simulink library "PhD_Library"  (R2018a)
settings: Solver=VariableStepAuto  StartTime=0.0  StopTime=10.0  RelTol=1e-3
values from neighbouring files (symbols this model uses):
  Ts = Ts_c    (= 1e-07)    [PlantStateEquations_abc_Script.m]
undefined symbols (not defined in the file or in its folder): D1, Delta, DiscIntNeverNeededParam, ESS, f_LPF_noise, fcutouti, fcutoutv, fn, fsw, Iap, Kp, PCC, Sn, tctrl, Ti, Ts_control, Ts_PWM, Uabp, Uanp, WT, X, zeta
libraries: $bdroot x84, powerlib_meascontrol x59, powerlib x56, peTransforms x32, cstblocks x2, simulink x2
(part 4 of 5)

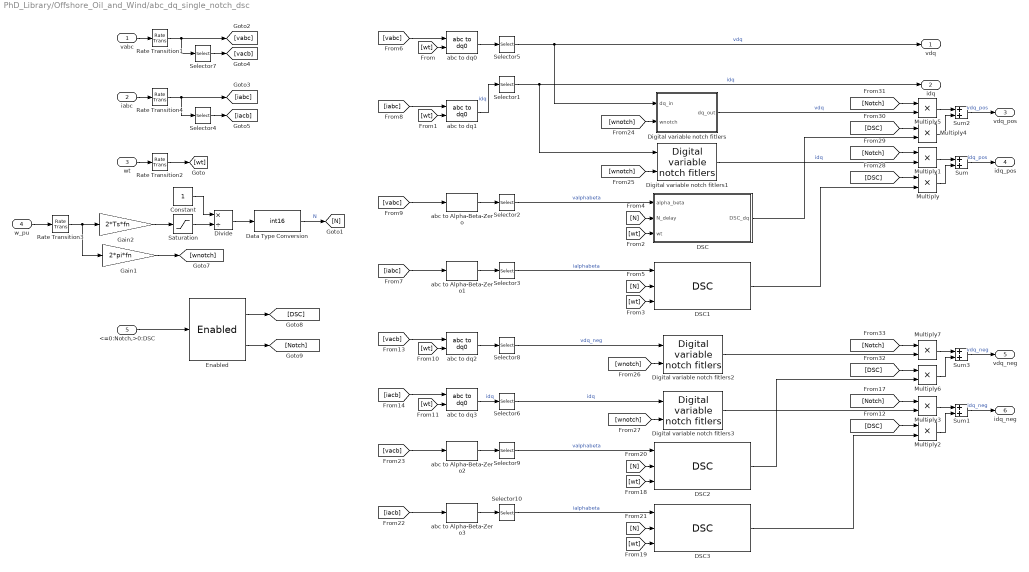
== system PhD_Library/Offshore_Oil_and_Wind/abc_dq_single_notch_dsc ==
  vabc : Inport
  iabc : Inport  Port=2
  wt : Inport  Port=3
  w_pu : Inport  Port=4
  <=0:Notch,>0:DSC : Inport  Port=5
  Constant : Constant
  DSC : Subsystem
  DSC1 : $bdroot/Offshore_Oil_and_Wind/abc_dq_single_notch_dsc/DSC
  DSC2 : $bdroot/Offshore_Oil_and_Wind/abc_dq_single_notch_dsc/DSC
  DSC3 : $bdroot/Offshore_Oil_and_Wind/abc_dq_single_notch_dsc/DSC
  Data Type Conversion : DataTypeConversion  OutDataTypeStr=int16  RndMeth=Round  SaturateOnIntegerOverflow=on
  Digital variable notch fitlers : Subsystem
  Digital variable notch fitlers1 : $bdroot/Offshore_Oil_and_Wind/abc_dq_single_notch_dsc/Digital variable notch fitlers
  Digital variable notch fitlers2 : $bdroot/Offshore_Oil_and_Wind/abc_dq_single_notch_dsc/Digital variable notch fitlers
  Digital variable notch fitlers3 : $bdroot/Offshore_Oil_and_Wind/abc_dq_single_notch_dsc/Digital variable notch fitlers
  Divide : Product  Inputs=*/
  Enabled : $bdroot/Offshore_Oil_and_Wind/Enabled
  Gain1 : Gain  Gain=2*pi*fn
  Gain2 : Gain  Gain=2*Ts*fn
  Multiply{,1..7} (8 alike) : Product
  Rate Transition1 : RateTransition  OutPortSampleTime=Ts
  Rate Transition2 : RateTransition  OutPortSampleTime=Ts
  Rate Transition3 : RateTransition  InitialCondition=1  OutPortSampleTime=Ts
  Rate Transition4 : RateTransition  OutPortSampleTime=Ts
  Saturation : Saturate  UpperLimit=inf  LowerLimit=0.000001
  Selector{1..3,5..6,8..10} (8 alike) : Selector  InputPortWidth=3  IndexOptions=Index vector (dialog)  Indices=[1 2]  OutputSizes=1
  Selector4 : Selector  InputPortWidth=3  IndexOptions=Index vector (dialog)  Indices=[1 3 2]  OutputSizes=1
  Selector7 : Selector  InputPortWidth=3  IndexOptions=Index vector (dialog)  Indices=[1 3 2]  OutputSizes=1
  Sum{,1..3} (4 alike) : Sum
  abc to Alpha-Beta-Zero{,1..3} (4 alike) : powerlib_meascontrol/Transformations/abc to Alpha-Beta-Zero
      settings: SourceProductName=Simscape Power Systems
  abc to dq{0..3} (4 alike) : powerlib_meascontrol/Transformations/abc to dq0  Alignment=90 degrees behind phase A axis
  vdq : Outport
  idq : Outport  Port=2
  vdq_pos : Outport  Port=3
  idq_pos : Outport  Port=4
  vdq_neg : Outport  Port=5
  idq_neg : Outport  Port=6
  wires:
  wt/1 -> Rate Transition2/1
  abc to dq1/1 -> Selector1/1  "idq"
  Selector5/1 -> Digital variable notch fitlers/1(dq_in), vdq/1  "vdq"
  abc to dq0/1 -> Selector5/1
  Selector1/1 -> Digital variable notch fitlers1/1, idq/1  "idq"
  abc to Alpha-Beta-Zero/1 -> Selector2/1
  abc to Alpha-Beta-Zero1/1 -> Selector3/1
  DSC/1(DSC_dq) -> Multiply4/2
  Selector3/1 -> DSC1/1  "ialphabeta"
  [vabc] -> abc to dq0/1
  [iabc] -> abc to dq1/1
  vabc/1 -> Rate Transition1/1
  iabc/1 -> Rate Transition4/1
  Selector2/1 -> DSC/1(alpha_beta)  "valphabeta"
  Digital variable notch fitlers/1(dq_out) -> Multiply5/2  "vdq"
  Digital variable notch fitlers1/1 -> Multiply1/2  "idq"
  DSC1/1 -> Multiply/2
  Sum2/1 -> vdq_pos/1  "vdq_pos"
  Sum/1 -> idq_pos/1  "idq_pos"
  Rate Transition2/1 -> [wt]
  [wt] -> abc to dq0/2
  [wt] -> abc to dq1/2
  [wt] -> DSC/3(wt)
  [wt] -> DSC1/3
  [N] -> DSC/2(N_delay)
  [N] -> DSC1/2
  Data Type Conversion/1 -> [N]  "N"
  Rate Transition1/1 -> Selector7/1, [vabc]
  Selector7/1 -> [vacb]
  Rate Transition4/1 -> Selector4/1, [iabc]
  Selector4/1 -> [iacb]
  [vabc] -> abc to Alpha-Beta-Zero/1
  [iabc] -> abc to Alpha-Beta-Zero1/1
  [wt] -> abc to dq3/2
  abc to dq2/1 -> Selector8/1
  Selector8/1 -> Digital variable notch fitlers2/1  "vdq_neg"
  [vacb] -> abc to dq2/1
  [wt] -> abc to dq2/2
  abc to dq3/1 -> Selector6/1  "idq"
  [iacb] -> abc to dq3/1
  Sum3/1 -> vdq_neg/1  "vdq_neg"
  Sum1/1 -> idq_neg/1  "idq_neg"
  Digital variable notch fitlers2/1 -> Multiply7/2
  Selector6/1 -> Digital variable notch fitlers3/1  "idq"
  Digital variable notch fitlers3/1 -> Multiply3/2
  abc to Alpha-Beta-Zero3/1 -> Selector10/1
  Selector10/1 -> DSC3/1  "ialphabeta"
  abc to Alpha-Beta-Zero2/1 -> Selector9/1
  [iacb] -> abc to Alpha-Beta-Zero3/1
  [wt] -> DSC2/3
  [vacb] -> abc to Alpha-Beta-Zero2/1
  DSC2/1 -> Multiply6/2
  Selector9/1 -> DSC2/1  "valphabeta"
  [N] -> DSC3/2
  [N] -> DSC2/2
  DSC3/1 -> Multiply2/2
  [wt] -> DSC3/3
  Gain2/1 -> Saturation/1
  Saturation/1 -> Divide/2
  Constant/1 -> Divide/1
  Rate Transition3/1 -> Gain1/1, Gain2/1
  Divide/1 -> Data Type Conversion/1
  w_pu/1 -> Rate Transition3/1
  Gain1/1 -> [wnotch]
  [wnotch] -> Digital variable notch fitlers/2(wnotch)
  [wnotch] -> Digital variable notch fitlers1/2
  [wnotch] -> Digital variable notch fitlers2/2
  [wnotch] -> Digital variable notch fitlers3/2
  <=0:Notch,>0:DSC/1 -> Enabled/1
  Enabled/1 -> [DSC]
  Enabled/2 -> [Notch]
  [DSC] -> Multiply/1
  [Notch] -> Multiply1/1
  Multiply1/1 -> Sum/1
  Multiply/1 -> Sum/2
  [Notch] -> Multiply3/1
  [DSC] -> Multiply2/1
  Multiply3/1 -> Sum1/1
  Multiply2/1 -> Sum1/2
  [Notch] -> Multiply5/1
  Multiply4/1 -> Sum2/2
  [DSC] -> Multiply4/1
  Multiply5/1 -> Sum2/1
  [Notch] -> Multiply7/1
  Multiply6/1 -> Sum3/2
  [DSC] -> Multiply6/1
  Multiply7/1 -> Sum3/1

== system PhD_Library/Offshore_Oil_and_Wind/abc_dq_with_AMA ==
  vabc : Inport
  iabc : Inport  Port=2
  wt : Inport  Port=3
  w_pu : Inport  Port=4
  AMA with retrieval pointer driven buffer{1..4} (4 alike) : $bdroot/Adaptive Moving Averages/AMA with retrieval pointer driven buffer  NbSize=1/(2*fmin*Ts)  Ts=Ts
  Bus Creator : BusCreator  Inputs=4
  Constant : Constant  Value=2*Ts
  Constant1 : Constant
  Demux : Demux  Outputs=2
  Demux1 : Demux  Outputs=2
  Digital first order LPF : $bdroot/Offshore_Oil_and_Wind/Digital first order LPF  Ts=Ts  fcutout=fcutoutv
  Digital first order LPF1 : $bdroot/Offshore_Oil_and_Wind/Digital first order LPF  Ts=Ts  fcutout=fcutouti
  Divide : Product  Inputs=*/
  Gain : Gain  Gain=fn
  Mux : Mux  Inputs=2
  Mux1 : Mux  Inputs=2
  Product : Product
  Rate Transition1 : RateTransition  OutPortSampleTime=Ts
  Rate Transition2 : RateTransition  OutPortSampleTime=Ts
  Rate Transition3 : RateTransition  InitialCondition=1  OutPortSampleTime=Ts
  Rate Transition4 : RateTransition  OutPortSampleTime=Ts
  Saturation : Saturate  UpperLimit=fmax  LowerLimit=fmin
  Selector4 : Selector  InputPortWidth=3  IndexOptions=Index vector (dialog)  Indices=[1 2]  OutputSizes=1
  Selector5 : Selector  InputPortWidth=3  IndexOptions=Index vector (dialog)  Indices=[1 2]  OutputSizes=1
  Terminator{1..8} (8 alike) : Terminator
  abc to dq0 : powerlib_meascontrol/Transformations/abc to dq0  Alignment=90 degrees behind phase A axis
  abc to dq1 : powerlib_meascontrol/Transformations/abc to dq0  Alignment=90 degrees behind phase A axis
  vdq : Outport
  idq : Outport  Port=2
  m : Outport  Port=3
  wires:
  Digital first order LPF/1 -> Demux/1  "vdq"
  abc to dq1/1 -> Selector4/1
  Mux1/1 -> Bus Creator/4, idq/1  "idq"
  Selector5/1 -> Digital first order LPF/1, Bus Creator/1  "vdq_unfilt"
  Rate Transition1/1 -> abc to dq0/1
  Rate Transition2/1 -> abc to dq0/2, abc to dq1/2
  Selector4/1 -> Bus Creator/2, Digital first order LPF1/1  "idq_unfilt"
  Rate Transition4/1 -> abc to dq1/1
  abc to dq0/1 -> Selector5/1
  Bus Creator/1 -> m/1
  Mux/1 -> Bus Creator/3, vdq/1  "vdq"
  wt/1 -> Rate Transition2/1
  vabc/1 -> Rate Transition1/1
  iabc/1 -> Rate Transition4/1
  AMA with retrieval pointer driven buffer1/3 -> Terminator2/1
  AMA with retrieval pointer driven buffer1/2 -> Terminator3/1
  w_pu/1 -> Rate Transition3/1
  Rate Transition3/1 -> Gain/1
  Gain/1 -> Saturation/1
  Saturation/1 -> Product/1
  Constant/1 -> Product/2
  Product/1 -> Divide/2
  Constant1/1 -> Divide/1
  Divide/1 -> [N]
  Demux/1 -> AMA with retrieval pointer driven buffer2/1
  Demux/2 -> AMA with retrieval pointer driven buffer1/1
  AMA with retrieval pointer driven buffer2/3 -> Terminator4/1
  AMA with retrieval pointer driven buffer2/2 -> Terminator5/1
  AMA with retrieval pointer driven buffer2/1 -> Mux/1
  AMA with retrieval pointer driven buffer1/1 -> Mux/2  "vdq"
  AMA with retrieval pointer driven buffer3/1 -> Mux1/2  "vdq"
  AMA with retrieval pointer driven buffer4/2 -> Terminator8/1
  Demux1/1 -> AMA with retrieval pointer driven buffer4/1
  Demux1/2 -> AMA with retrieval pointer driven buffer3/1
  AMA with retrieval pointer driven buffer4/3 -> Terminator7/1
  AMA with retrieval pointer driven buffer3/3 -> Terminator1/1
  AMA with retrieval pointer driven buffer4/1 -> Mux1/1
  AMA with retrieval pointer driven buffer3/2 -> Terminator6/1
  Digital first order LPF1/1 -> Demux1/1  "idq"
  [N] -> AMA with retrieval pointer driven buffer2/2
  [N] -> AMA with retrieval pointer driven buffer1/2
  [N] -> AMA with retrieval pointer driven buffer4/2
  [N] -> AMA with retrieval pointer driven buffer3/2

== system PhD_Library/Offshore_Oil_and_Wind/abc_dq_with_PLL ==
  vabc : Inport
  iabc : Inport  Port=2
  Bus Creator : BusCreator  Inputs=4
  PLL (3ph) : powerlib_meascontrol/PLL/PLL (3ph)  Fmin=0.8*fn  Par_Init=[0, fn]  ParK=[Kp_pll, Ki_pll, Kd_pll]  TcD=1e-4  MaxRateChangeFreq=fn/5  FilterCutOffFreq=fn/2  Ts=Ts  AGC=on
  Rate Transition1 : RateTransition  OutPortSampleTime=Ts
  Rate Transition4 : RateTransition  OutPortSampleTime=Ts
  Rtot_pu3 : Gain  Gain=1/fn  SaturateOnIntegerOverflow=on  OutDataTypeStr=Inherit: Same as input  ParamDataTypeStr=Inherit: Same as input
  Second-Order Filter1 : powerlib_meascontrol/Filters/Second-Order Filter  FilterType=Bandstop (Notch)  Fo=fn  Zeta=zeta  Ts=Ts  Initialize=off  Vac_Init="[0,  0,  60]"  Vdc_Init=0  PlotResponse=off  FreqRange=[0, 1000, 0.1]
      settings: SourceProductName=Simscape Power Systems  SourceProductBaseCode=PS
  Second-Order Filter2 : powerlib_meascontrol/Filters/Second-Order Filter  FilterType=Lowpass  Fo=fcutoutv  Zeta=zeta  Ts=Ts  Initialize=off  Vac_Init="[0,  0,  60]"  Vdc_Init=0  PlotResponse=off  FreqRange=[0, 1000, 0.1]
      settings: SourceProductName=Simscape Power Systems  SourceProductBaseCode=PS
  Second-Order Filter3 : powerlib_meascontrol/Filters/Second-Order Filter  FilterType=Lowpass  Fo=fcutouti  Zeta=zeta  Ts=Ts  Initialize=off  Vac_Init="[0,  0,  60]"  Vdc_Init=0  PlotResponse=off  FreqRange=[0, 1000, 0.1]
      settings: SourceProductName=Simscape Power Systems  SourceProductBaseCode=PS
  Second-Order Filter5 : powerlib_meascontrol/Filters/Second-Order Filter  FilterType=Bandstop (Notch)  Fo=fn  Zeta=zeta  Ts=Ts  Initialize=off  Vac_Init="[0,  0,  60]"  Vdc_Init=0  PlotResponse=off  FreqRange=[0, 1000, 0.1]
      settings: SourceProductName=Simscape Power Systems  SourceProductBaseCode=PS
  Selector4 : Selector  InputPortWidth=3  IndexOptions=Index vector (dialog)  Indices=[1 2]  OutputSizes=1
  Selector5 : Selector  InputPortWidth=3  IndexOptions=Index vector (dialog)  Indices=[1 2]  OutputSizes=1
  abc to dq0 : powerlib_meascontrol/Transformations/abc to dq0  Alignment=90 degrees behind phase A axis
  abc to dq1 : powerlib_meascontrol/Transformations/abc to dq0  Alignment=90 degrees behind phase A axis
  vdq : Outport
  idq : Outport  Port=2
  f_pu : Outport  Port=3
  wt : Outport  Port=4
  m : Outport  Port=5
  wires:
  Rtot_pu3/1 -> f_pu/1
  Second-Order Filter3/1 -> Second-Order Filter1/1
  Second-Order Filter2/1 -> Second-Order Filter5/1  "vdq"
  abc to dq1/1 -> Selector4/1
  Second-Order Filter1/1 -> Bus Creator/4, idq/1  "idq"
  vabc/1 -> Rate Transition1/1
  Selector5/1 -> Second-Order Filter2/1, Bus Creator/1  "vdq_unfilt"
  Rate Transition1/1 -> abc to dq0/1, PLL (3ph)/1
  iabc/1 -> Rate Transition4/1
  PLL (3ph)/2 -> wt/1, abc to dq1/2, abc to dq0/2
  Selector4/1 -> Second-Order Filter3/1, Bus Creator/2  "idq_unfilt"
  Rate Transition4/1 -> abc to dq1/1
  abc to dq0/1 -> Selector5/1
  PLL (3ph)/1 -> Rtot_pu3/1
  Bus Creator/1 -> m/1
  Second-Order Filter5/1 -> vdq/1, Bus Creator/3  "vdq"

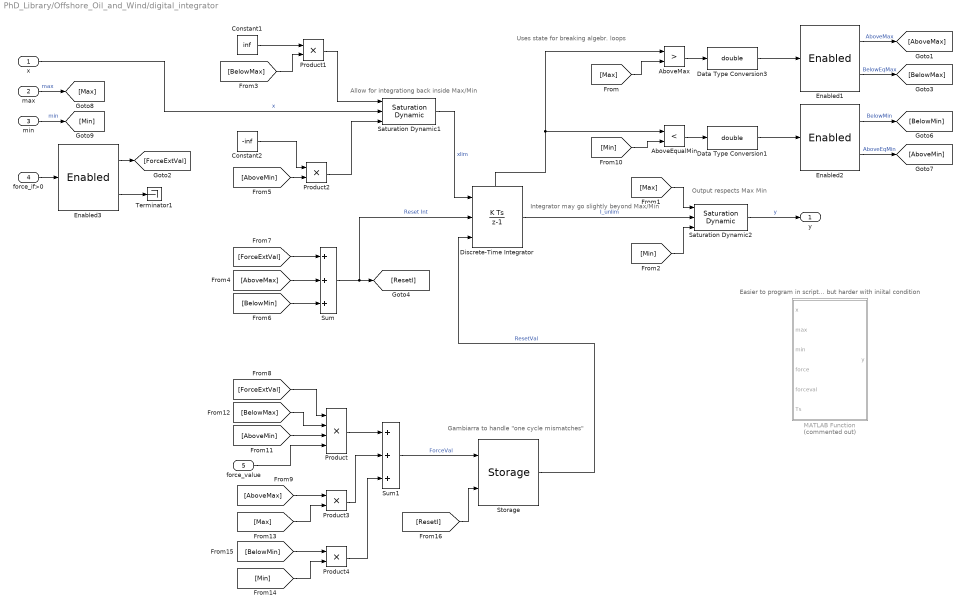
== system PhD_Library/Offshore_Oil_and_Wind/digital_integrator ==
  note: Gambiarra to handle "one cycle mismatches"
  note: Integrator may go slightly beyond Max/Min
  note: Output respects Max Min
  note: Uses state for breaking algebr. loops
  note: Allow for integrationg back inside Max/Min
  note: Easier to program in script... but harder with iniital condition
  x : Inport
  max : Inport  Port=2
  min : Inport  Port=3
  force_if>0 : Inport  Port=4
  force_value : Inport  Port=5
  AboveEqualMin : RelationalOperator  Operator=<  OutDataTypeStr=boolean  RndMeth=Simplest
  AboveMax : RelationalOperator  Operator=>  OutDataTypeStr=boolean  RndMeth=Simplest
  Constant1 : Constant  Value=inf
  Constant2 : Constant  Value=-inf
  Data Type Conversion1 : DataTypeConversion  OutDataTypeStr=double
  Data Type Conversion3 : DataTypeConversion  OutDataTypeStr=double
  Discrete-Time Integrator : DiscreteIntegrator  ExternalReset=level  InitialConditionSource=external  SampleTime=Ts  ShowStatePort=on  IgnoreLimit=on  ICPrevOutput=DiscIntNeverNeededParam  ICPrevScaledInput=DiscIntNeverNeededParam
  Enabled1 : $bdroot/Offshore_Oil_and_Wind/Enabled
  Enabled2 : $bdroot/Offshore_Oil_and_Wind/Enabled
  Enabled3 : $bdroot/Offshore_Oil_and_Wind/Enabled
  MATLAB Function : MATLAB Function  Commented=on  TreatAsAtomicUnit=on  SystemSampleTime=Ts
      settings: RTWSystemCode=Inline
  Product : Product  Inputs=4
  Product{1..4} (4 alike) : Product
  Saturation Dynamic1 : simulink/Discontinuities/Saturation Dynamic  OutMin=[]  OutMax=[]  OutDataTypeStr=Inherit: Same as second input  OutDataType=fixdt(1, 16)  OutScaling=2^-10  DoSatur=off
  Saturation Dynamic2 : simulink/Discontinuities/Saturation Dynamic  OutMin=[]  OutMax=[]  OutDataTypeStr=Inherit: Same as second input  OutDataType=fixdt(1, 16)  OutScaling=2^-10  DoSatur=off
  Storage : $bdroot/Offshore_Oil_and_Wind/Storage
  Sum : Sum  Inputs=+++
  Sum1 : Sum  Inputs=+++
  Terminator1 : Terminator
  y : Outport
  wires:
  x/1 -> Saturation Dynamic1/2  "x"
  Saturation Dynamic2/1 -> y/1  "y"
  max/1 -> [Max]  "max"
  min/1 -> [Min]  "min"
  force_value/1 -> Product/4
  Saturation Dynamic1/1 -> Discrete-Time Integrator/1  "xlim"
  [BelowMax] -> Product1/2
  Constant1/1 -> Product1/1
  Product1/1 -> Saturation Dynamic1/1
  [AboveMin] -> Product2/2
  Constant2/1 -> Product2/1
  Product2/1 -> Saturation Dynamic1/3
  Enabled1/1 -> [AboveMax]  "AboveMax"
  Enabled1/2 -> [BelowMax]  "BelowEqMax"
  Enabled2/2 -> [AboveMin]  "AboveEqMin"
  Enabled2/1 -> [BelowMin]  "BelowMin"
  [AboveMax] -> Sum/2
  [BelowMin] -> Sum/3
  force_if>0/1 -> Enabled3/1
  Enabled3/2 -> Terminator1/1
  [ForceExtVal] -> Product/1
  [AboveMax] -> Product3/1
  [Min] -> AboveEqualMin/2
  [AboveMin] -> Product/3
  [BelowMax] -> Product/2
  Product/1 -> Sum1/1
  [Max] -> Product3/2
  [BelowMin] -> Product4/1
  [Min] -> Product4/2
  Product4/1 -> Sum1/3
  Product3/1 -> Sum1/2
  Sum1/1 -> Storage/1  "ForceVal"
  Enabled3/1 -> [ForceExtVal]
  [Max] -> AboveMax/2
  Discrete-Time Integrator/1 -> Saturation Dynamic2/2  "I_unlim"
  [Max] -> Saturation Dynamic2/1
  [Min] -> Saturation Dynamic2/3
  AboveMax/1 -> Data Type Conversion3/1
  AboveEqualMin/1 -> Data Type Conversion1/1
  Data Type Conversion3/1 -> Enabled1/1
  Data Type Conversion1/1 -> Enabled2/1
  [ForceExtVal] -> Sum/1
  Discrete-Time Integrator/State -> AboveEqualMin/1, AboveMax/1
  Sum/1 -> Discrete-Time Integrator/2, [ResetI]  "Reset Int"
  [ResetI] -> Storage/2
  Storage/1 -> Discrete-Time Integrator/3  "ResetVal"

== system PhD_Library/Offshore_Oil_and_Wind/digital_ramp_gen ==
  up_if>0 : Inport
  down_if>0 : Inport  Port=2
  rate_pu/s : Inport  Port=3
  max : Inport  Port=4
  min : Inport  Port=5
  force_if=1 : Inport  Port=6
  force_value : Inport  Port=7
  Constant : Constant  Value=Ts
  MATLAB Function : MATLAB Function  TreatAsAtomicUnit=on  SystemSampleTime=Ts
      settings: RTWSystemCode=Inline
  y : Outport
  wires:
  up_if>0/1 -> MATLAB Function/1(up)
  MATLAB Function/1(y) -> y/1
  max/1 -> MATLAB Function/4(max)
  min/1 -> MATLAB Function/5(min)
  force_if=1/1 -> MATLAB Function/6(force)
  force_value/1 -> MATLAB Function/7(forceval)
  Constant/1 -> MATLAB Function/8(Ts)
  down_if>0/1 -> MATLAB Function/2(down)
  rate_pu/s/1 -> MATLAB Function/3(rate)

== system PhD_Library/Offshore_Oil_and_Wind/idqref_gen_for_cnst_p ==
  vdq+ : Inport
  vdq- : Inport  Port=2
  idqref : Inport  Port=3
  MATLAB Function : MATLAB Function  TreatAsAtomicUnit=on  SystemSampleTime=Ts
  idqref- : Outport
  wires:
  MATLAB Function/1(idqref) -> idqref-/1
  vdq+/1 -> MATLAB Function/1(vdqp)
  vdq-/1 -> MATLAB Function/2(vdqn)
  idqref/1 -> MATLAB Function/3("idqref ")

== system PhD_Library/Offshore_Oil_and_Wind/idref_gen ==
  vdq+ : Inport
  vdq- : Inport  Port=2
  idref : Inport  Port=3
  Add : Sum
  Add1 : Sum
  Constant : Constant
  Demux : Demux  Outputs=2
  Demux1 : Demux  Outputs=2
  Divide : Product  Inputs=*/
  Gain : Gain  Gain=-1
  Gain1 : Gain  Gain=-1
  Mux : Mux  Inputs=2
  Mux1 : Mux  Inputs=2
  Product{,2,4..5} (4 alike) : Product
  Product{1,3,6..7} (4 alike) : Product  Inputs=3
  Saturation : Saturate  UpperLimit=inf  LowerLimit=0.000001
  Subtract : Sum  Inputs=+-
  idqref+ : Outport
  idqref- : Outport  Port=2
  wires:
  Product/1 -> Add/1
  Product2/1 -> Add/2
  Add/1 -> Subtract/1
  Add1/1 -> Subtract/2
  Product4/1 -> Add1/1
  Product5/1 -> Add1/2
  Demux/1 -> Product1/2, Product/1, Product/2
  Demux/2 -> Product3/2, Product2/2, Product2/1
  Demux1/1 -> Gain/1, Product4/2, Product4/1
  Gain/1 -> Product6/2
  idref/1 -> Product1/1, Product3/1, Product6/1, Product7/1
  Demux1/2 -> Gain1/1, Product5/1, Product5/2
  Gain1/1 -> Product7/2
  Subtract/1 -> Saturation/1
  Divide/1 -> [D]
  Constant/1 -> Divide/1
  [D] -> Product1/3
  [D] -> Product3/3
  [D] -> Product6/3
  [D] -> Product7/3
  Product1/1 -> Mux/1
  Product3/1 -> Mux/2
  Mux/1 -> idqref+/1
  Product6/1 -> Mux1/1
  Mux1/1 -> idqref-/1
  Product7/1 -> Mux1/2
  vdq+/1 -> Demux/1
  vdq-/1 -> Demux1/1
  Saturation/1 -> Divide/2

== system PhD_Library/Offshore_Oil_and_Wind/pqui_Transd_DSC ==
  Vabc : Inport
  Iabc : Inport  Port=2
  w_pu : Inport  Port=3
  Clarke Transform{,1..3} (4 alike) : peTransforms/Clarke Transform  PowerInvariant=off
  DSC_Neg : $bdroot/Offshore_Oil_and_Wind/pqui_Transd_DSC/DSC_Pos 
  "DSC_Pos " : Subsystem
  Data Type Conversion : DataTypeConversion  OutDataTypeStr=int16  RndMeth=Round  SaturateOnIntegerOverflow=on
  Gain6 : Gain  Gain=1/(4*Ts*fn)
  PQVI : Subsystem
  PQVI_Neg : $bdroot/Offshore_Oil_and_Wind/pqui_Transd_DSC/PQVI
  PQVI_Pos : $bdroot/Offshore_Oil_and_Wind/pqui_Transd_DSC/PQVI
  Rate Transition1 : RateTransition  OutPortSampleTime=Ts
  Rate Transition3 : RateTransition  InitialCondition=1  OutPortSampleTime=Ts
  Rate Transition5 : RateTransition  OutPortSampleTime=Ts
  Selector{1,4..6} (4 alike) : Selector  InputPortWidth=3  IndexOptions=Index vector (dialog)  Indices=[1 2]  OutputSizes=1
  Selector2 : Selector  InputPortWidth=3  IndexOptions=Index vector (dialog)  Indices=[1 3 2]  OutputSizes=1
  Selector3 : Selector  InputPortWidth=3  IndexOptions=Index vector (dialog)  Indices=[1 3 2]  OutputSizes=1
  pqvi : Outport
  pqvi+ : Outport  Port=2
  pqvi- : Outport  Port=3
  wires:
  Clarke Transform1/1 -> Selector1/1
  Vabc/1 -> Rate Transition1/1
  Clarke Transform/1 -> Selector5/1
  Iabc/1 -> Rate Transition5/1
  w_pu/1 -> Rate Transition3/1
  Rate Transition1/1 -> Selector2/1, Clarke Transform/1
  Rate Transition5/1 -> Selector3/1, Clarke Transform1/1
  Selector5/1 -> "DSC_Pos "/1(valphabeta), PQVI/1(valphabeta)
  Selector1/1 -> "DSC_Pos "/2(ialphabeta), PQVI/2(ialphabeta)
  PQVI/1(pqvi) -> pqvi/1
  Rate Transition3/1 -> Gain6/1
  Data Type Conversion/1 -> DSC_Neg/3, "DSC_Pos "/3(Nsamp_delay)
  Gain6/1 -> Data Type Conversion/1
  "DSC_Pos "/1(valphabeta_DSC) -> PQVI_Pos/1
  "DSC_Pos "/2(ialphabeta_DSC) -> PQVI_Pos/2
  PQVI_Pos/1 -> pqvi+/1
  Clarke Transform2/1 -> Selector6/1
  Clarke Transform3/1 -> Selector4/1
  Selector2/1 -> Clarke Transform2/1
  Selector3/1 -> Clarke Transform3/1
  Selector6/1 -> DSC_Neg/1
  Selector4/1 -> DSC_Neg/2
  PQVI_Neg/1 -> pqvi-/1
  DSC_Neg/2 -> PQVI_Neg/2
  DSC_Neg/1 -> PQVI_Neg/1

== system PhD_Library/Offshore_Oil_and_Wind/pqui_Transd_NoZeroSeq ==
  note: Akagi 1984 for p and q
      | calc. without zero seq,
      | factor 3/2 compensates for
      | amplitude invariant
      | Clarke transformation
  Vabc : Inport
  Iabc : Inport  Port=2
  Add3 : Sum  Inputs=+-
  Clarke Transform : peTransforms/Clarke Transform  PowerInvariant=off
  Clarke Transform1 : peTransforms/Clarke Transform  PowerInvariant=off
  Demux1 : Demux  Outputs=2
  Demux4 : Demux  Outputs=2
  Dot Product : DotProduct  InputSameDT=on  OutDataTypeStr=Inherit: Inherit via internal rule
  Gain1 : Gain  Gain=3/2/Sn
  Gain2 : Gain  Gain=3/2/Sn
  Gain3 : Gain  Gain=1/Uanp
  Gain4 : Gain  Gain=1/Iap
  Hypot : Math  Operator=hypot  RndMeth=Zero  SaturateOnIntegerOverflow=on
  Hypot1 : Math  Operator=hypot  RndMeth=Zero  SaturateOnIntegerOverflow=on
  Product3 : Product
  Product4 : Product
  Selector1 : Selector  InputPortWidth=3  IndexOptions=Index vector (dialog)  Indices=[1 2]  OutputSizes=1
  Selector5 : Selector  InputPortWidth=3  IndexOptions=Index vector (dialog)  Indices=[1 2]  OutputSizes=1
  p : Outport
  q : Outport  Port=2
  v : Outport  Port=3
  i : Outport  Port=4
  wires:
  Clarke Transform1/1 -> Selector1/1
  Gain3/1 -> v/1  "v"
  Demux1/2 -> Hypot1/2, Product4/2
  Hypot1/1 -> Gain4/1  "i"
  Selector1/1 -> Demux1/1, Dot Product/2
  Selector5/1 -> Demux4/1, Dot Product/1
  Demux4/1 -> Hypot/1, Product4/1
  Hypot/1 -> Gain3/1  "v"
  Dot Product/1 -> Gain1/1  "p"
  Demux1/1 -> Hypot1/1, Product3/2
  Add3/1 -> Gain2/1  "q"
  Product4/1 -> Add3/2
  Demux4/2 -> Hypot/2, Product3/1
  Vabc/1 -> Clarke Transform/1
  Clarke Transform/1 -> Selector5/1
  Iabc/1 -> Clarke Transform1/1
  Product3/1 -> Add3/1
  Gain1/1 -> p/1  "p"
  Gain4/1 -> i/1  "i"
  Gain2/1 -> q/1  "q"

== system PhD_Library/Offshore_Oil_and_Wind/pqui_Transd_NoZeroSeq_Filter ==
  note: Akagi 1984 for p and q
      | calc. without zero seq,
      | factor 3/2 compensates for
      | amplitude invariant
      | Clarke transformation
  Vabc : Inport
  Iabc : Inport  Port=2
  Add3 : Sum  Inputs=+-
  Clarke Transform : peTransforms/Clarke Transform  PowerInvariant=off
  Clarke Transform1 : peTransforms/Clarke Transform  PowerInvariant=off
  Demux1 : Demux  Outputs=2
  Demux4 : Demux  Outputs=2
  Dot Product : DotProduct  InputSameDT=on  OutDataTypeStr=Inherit: Inherit via internal rule
  Gain1 : Gain  Gain=3/2/Sn
  Gain2 : Gain  Gain=3/2/Sn
  Gain3 : Gain  Gain=1/Uanp
  Gain4 : Gain  Gain=1/Iap
  Hypot : Math  Operator=hypot  RndMeth=Zero  SaturateOnIntegerOverflow=on
  Hypot1 : Math  Operator=hypot  RndMeth=Zero  SaturateOnIntegerOverflow=on
  Product3 : Product
  Product4 : Product
  Rate Transition1 : RateTransition  OutPortSampleTime=Ts
  Rate Transition2 : RateTransition  OutPortSampleTime=Ts
  Second-Order Filter1 : powerlib_meascontrol/Filters/Second-Order Filter  FilterType=Lowpass  Fo=fcutoutvi  Zeta=zeta  Ts=Ts  Initialize=off  Vac_Init="[0,  0,  60]"  Vdc_Init=0  PlotResponse=off  FreqRange=[0, 1000, 0.1]
      settings: SourceProductName=Simscape Power Systems  SourceProductBaseCode=PS
  Second-Order Filter2 : powerlib_meascontrol/Filters/Second-Order Filter  FilterType=Lowpass  Fo=fcutoutvi  Zeta=zeta  Ts=Ts  Initialize=off  Vac_Init="[0,  0,  60]"  Vdc_Init=0  PlotResponse=off  FreqRange=[0, 1000, 0.1]
      settings: SourceProductName=Simscape Power Systems  SourceProductBaseCode=PS
  Second-Order Filter{3,5..6,8} (4 alike) : powerlib_meascontrol/Filters/Second-Order Filter  FilterType=Bandstop (Notch)  Fo=fn  Zeta=zeta  Ts=Ts  Initialize=off  Vac_Init="[0,  0,  60]"  Vdc_Init=0  PlotResponse=off  FreqRange=[0, 1000, 0.1]
      settings: SourceProductName=Simscape Power Systems  SourceProductBaseCode=PS
  Second-Order Filter4 : powerlib_meascontrol/Filters/Second-Order Filter  FilterType=Lowpass  Fo=fcutoutpq  Zeta=zeta  Ts=Ts  Initialize=off  Vac_Init="[0,  0,  60]"  Vdc_Init=0  PlotResponse=off  FreqRange=[0, 1000, 0.1]
      settings: SourceProductName=Simscape Power Systems  SourceProductBaseCode=PS
  Second-Order Filter7 : powerlib_meascontrol/Filters/Second-Order Filter  FilterType=Lowpass  Fo=fcutoutpq  Zeta=zeta  Ts=Ts  Initialize=off  Vac_Init="[0,  0,  60]"  Vdc_Init=0  PlotResponse=off  FreqRange=[0, 1000, 0.1]
      settings: SourceProductName=Simscape Power Systems  SourceProductBaseCode=PS
  Selector1 : Selector  InputPortWidth=3  IndexOptions=Index vector (dialog)  Indices=[1 2]  OutputSizes=1
  Selector5 : Selector  InputPortWidth=3  IndexOptions=Index vector (dialog)  Indices=[1 2]  OutputSizes=1
  p : Outport
  q : Outport  Port=2
  v : Outport  Port=3
  i : Outport  Port=4
  wires:
  Clarke Transform1/1 -> Selector1/1
  Gain3/1 -> Second-Order Filter2/1  "v"
  Demux1/2 -> Hypot1/2, Product4/2
  Hypot1/1 -> Gain4/1  "i"
  Selector1/1 -> Demux1/1, Dot Product/2
  Selector5/1 -> Demux4/1, Dot Product/1
  Demux4/1 -> Hypot/1, Product4/1
  Hypot/1 -> Gain3/1  "v"
  Iabc/1 -> Rate Transition2/1
  Dot Product/1 -> Gain1/1  "p"
  Demux1/1 -> Hypot1/1, Product3/2
  Add3/1 -> Gain2/1  "q"
  Vabc/1 -> Rate Transition1/1
  Product4/1 -> Add3/2
  Demux4/2 -> Hypot/2, Product3/1
  Rate Transition1/1 -> Clarke Transform/1
  Clarke Transform/1 -> Selector5/1
  Rate Transition2/1 -> Clarke Transform1/1
  Product3/1 -> Add3/1
  Gain1/1 -> Second-Order Filter7/1  "p"
  Gain4/1 -> Second-Order Filter1/1  "i"
  Gain2/1 -> Second-Order Filter4/1  "q"
  Second-Order Filter2/1 -> Second-Order Filter5/1
  Second-Order Filter5/1 -> v/1
  Second-Order Filter1/1 -> Second-Order Filter3/1
  Second-Order Filter3/1 -> i/1
  Second-Order Filter4/1 -> Second-Order Filter6/1
  Second-Order Filter6/1 -> q/1
  Second-Order Filter8/1 -> p/1
  Second-Order Filter7/1 -> Second-Order Filter8/1

== system PhD_Library/Offshore_Oil_and_Wind/LSC_LCL_Trafo/INV_DClink ==
  CM : powerlib/Measurements/Current Measurement  PhasorSimulation=off  OutputType=Complex  PSBequivalent=0
  VM1 : powerlib/Measurements/Voltage Measurement  PhasorSimulation=off  OutputType=Complex  PSBequivalent=0
  Pin : PMIOPort  Side=Left
  Min : PMIOPort  Port=2  Side=Left
  Pout : PMIOPort  Port=3  Side=Right
  Mout : PMIOPort  Port=4  Side=Right
  Vdc : Outport
  Idc : Outport  Port=2
  wires:
  CM/1 -> Idc/1
  VM1/1 -> Vdc/1
  connections:
  VM1/LConn2 -- Mout/RConn1 -- Min/RConn1
  VM1/LConn1 -- CM/LConn1 -- Pin/RConn1
  CM/RConn1 -- Pout/RConn1

== system PhD_Library/Offshore_Oil_and_Wind/LSC_LCL_Trafo_AvgxSwitch/INV_DClink ==
  CM : powerlib/Measurements/Current Measurement  PhasorSimulation=off  OutputType=Complex  PSBequivalent=0
  VM1 : powerlib/Measurements/Voltage Measurement  PhasorSimulation=off  OutputType=Complex  PSBequivalent=0
  Pin : PMIOPort  Side=Left
  Min : PMIOPort  Port=2  Side=Left
  Pout : PMIOPort  Port=3  Side=Right
  Mout : PMIOPort  Port=4  Side=Right
  Vdc : Outport
  Idc : Outport  Port=2
  wires:
  CM/1 -> Idc/1
  VM1/1 -> Vdc/1
  connections:
  VM1/LConn2 -- Mout/RConn1 -- Min/RConn1
  VM1/LConn1 -- CM/LConn1 -- Pin/RConn1
  CM/RConn1 -- Pout/RConn1

== system PhD_Library/Offshore_Oil_and_Wind/abc_dq_single_notch_dsc/DSC ==
  note: 0+j1
  note: Delayed alpha beta zero
  alpha_beta : Inport
  N_delay : Inport  Port=2
  wt : Inport  Port=3
  Alpha-Beta-Zero to dq0 : powerlib_meascontrol/Transformations/Alpha-Beta-Zero to dq0  Alignment=90 degrees behind phase A axis
      settings: SourceProductName=Simscape Power Systems
  Complex to Real-Imag : ComplexToRealImag
  Constant1 : Constant  Value=0
  Constant3 : Constant  Value=0
  Constant4 : Constant
  Demux : Demux  Outputs=2
  Demux1 : Demux  Outputs=2
  Gain : Gain  Gain=0.5
  Mux1 : Mux  Inputs=[1 1 1]
  Product : Product
  Real-Imag to Complex : RealImagToComplex
  Real-Imag to Complex1 : RealImagToComplex
  Real-Imag to Complex2 : RealImagToComplex
  Selector4 : Selector  InputPortWidth=3  IndexOptions=Index vector (dialog)  Indices=[1 2]  OutputSizes=1
  Subtract : Sum
  Variable Integer Delay : Delay  DelayLengthSource=Input port  DelayLength=200  DelayLengthUpperLimit=500  SampleTime=Ts
      settings: InputPortMap=u0,p1
  DSC_dq : Outport
  wires:
  Product/1 -> Subtract/2
  Demux/1 -> Real-Imag to Complex/1
  Real-Imag to Complex1/1 -> Product/1
  Demux1/1 -> Real-Imag to Complex1/1
  wt/1 -> Alpha-Beta-Zero to dq0/2
  Complex to Real-Imag/1 -> Mux1/1
  Variable Integer Delay/1 -> Demux1/1
  Demux1/2 -> Real-Imag to Complex1/2
  N_delay/1 -> Variable Integer Delay/2
  Gain/1 -> Alpha-Beta-Zero to dq0/1
  Constant3/1 -> Real-Imag to Complex2/1
  Real-Imag to Complex/1 -> Subtract/1
  alpha_beta/1 -> Variable Integer Delay/1, Demux/1
  Real-Imag to Complex2/1 -> Product/2
  Subtract/1 -> Complex to Real-Imag/1
  Constant1/1 -> Mux1/3
  Demux/2 -> Real-Imag to Complex/2
  Constant4/1 -> Real-Imag to Complex2/2
  Complex to Real-Imag/2 -> Mux1/2
  Mux1/1 -> Gain/1
  Alpha-Beta-Zero to dq0/1 -> Selector4/1
  Selector4/1 -> DSC_dq/1

== system PhD_Library/Offshore_Oil_and_Wind/abc_dq_single_notch_dsc/Digital variable notch fitlers ==
  dq_in : Inport
  wnotch : Inport  Port=2
  Constant : Constant  Value=0
  Constant1 : Constant  Value=zeta
  Constant2 : Constant  Value=0
  Constant3 : Constant  Value=zeta
  Demux : Demux  Outputs=2
  Discrete Varying Notch : cstblocks/Linear Parameter Varying/Discrete Varying Notch  w0=0  Ts=Ts
      settings: SourceProductName=Control System Toolbox  SourceProductBaseCode=CT
  Discrete Varying Notch1 : cstblocks/Linear Parameter Varying/Discrete Varying Notch  w0=0  Ts=Ts
      settings: SourceProductName=Control System Toolbox  SourceProductBaseCode=CT
  Mux : Mux  Inputs=2
  dq_out : Outport
  wires:
  Constant/1 -> Discrete Varying Notch/3
  Constant1/1 -> Discrete Varying Notch/4
  Demux/2 -> Discrete Varying Notch1/1
  dq_in/1 -> Demux/1
  Constant2/1 -> Discrete Varying Notch1/3
  wnotch/1 -> Discrete Varying Notch1/2, Discrete Varying Notch/2
  Constant3/1 -> Discrete Varying Notch1/4
  Demux/1 -> Discrete Varying Notch/1
  Discrete Varying Notch/1 -> Mux/1
  Mux/1 -> dq_out/1
  Discrete Varying Notch1/1 -> Mux/2

== system PhD_Library/Offshore_Oil_and_Wind/pqui_Transd_DSC/DSC_Pos  ==
  valphabeta : Inport
  ialphabeta : Inport  Port=2
  Nsamp_delay : Inport  Port=3
  Complex to Real-Imag : ComplexToRealImag
  Complex to Real-Imag1 : ComplexToRealImag
  Constant3 : Constant  Value=0
  Constant4 : Constant
  Constant5 : Constant  Value=0
  Constant6 : Constant
  Demux{,2..3,5} (4 alike) : Demux  Outputs=2
  Gain : Gain  Gain=0.5
  Gain1 : Gain  Gain=0.5
  Mux1 : Mux  Inputs=[1 1]
  Mux2 : Mux  Inputs=[1 1]
  Product : Product
  Product1 : Product
  Real-Imag to Complex{,1..5} (6 alike) : RealImagToComplex
  Subtract : Sum
  Subtract1 : Sum
  Variable Integer Delay : Delay  DelayLengthSource=Input port  DelayLength=200  DelayLengthUpperLimit=500  SampleTime=Ts
      settings: InputPortMap=u0,p1
  Variable Integer Delay1 : Delay  DelayLengthSource=Input port  DelayLength=200  DelayLengthUpperLimit=500  SampleTime=Ts
      settings: InputPortMap=u0,p1
  valphabeta_DSC : Outport
  ialphabeta_DSC : Outport  Port=2
  wires:
  Demux2/2 -> Real-Imag to Complex1/2
  Demux3/1 -> Real-Imag to Complex3/1
  Constant6/1 -> Real-Imag to Complex5/2
  Constant5/1 -> Real-Imag to Complex5/1
  Real-Imag to Complex5/1 -> Product1/2
  Complex to Real-Imag1/1 -> Mux2/1
  Real-Imag to Complex4/1 -> Product1/1
  Demux3/2 -> Real-Imag to Complex3/2
  Gain1/1 -> ialphabeta_DSC/1  "ialphabeta"
  Complex to Real-Imag1/2 -> Mux2/2
  Complex to Real-Imag/1 -> Mux1/1
  Mux2/1 -> Gain1/1
  valphabeta/1 -> Demux/1, Variable Integer Delay/1
  Real-Imag to Complex2/1 -> Product/2
  Subtract1/1 -> Complex to Real-Imag1/1
  Real-Imag to Complex3/1 -> Subtract1/1
  Mux1/1 -> Gain/1
  Constant3/1 -> Real-Imag to Complex2/1
  Demux/1 -> Real-Imag to Complex/1
  Variable Integer Delay1/1 -> Demux5/1
  Demux5/2 -> Real-Imag to Complex4/2
  Demux2/1 -> Real-Imag to Complex1/1
  Variable Integer Delay/1 -> Demux2/1
  Product/1 -> Subtract/2
  Nsamp_delay/1 -> Variable Integer Delay1/2, Variable Integer Delay/2
  Complex to Real-Imag/2 -> Mux1/2
  Product1/1 -> Subtract1/2
  Gain/1 -> valphabeta_DSC/1  "valphabeta"
  Real-Imag to Complex1/1 -> Product/1
  Real-Imag to Complex/1 -> Subtract/1
  Subtract/1 -> Complex to Real-Imag/1
  Constant4/1 -> Real-Imag to Complex2/2
  ialphabeta/1 -> Demux3/1, Variable Integer Delay1/1
  Demux5/1 -> Real-Imag to Complex4/1
  Demux/2 -> Real-Imag to Complex/2

== system PhD_Library/Offshore_Oil_and_Wind/pqui_Transd_DSC/PQVI ==
  note: Akagi 1984 for p and q
      | calc. without zero seq,
      | factor 3/2 compensates for
      | amplitude invariant
      | Clarke transformation
  valphabeta : Inport
  ialphabeta : Inport  Port=2
  Add3 : Sum  Inputs=+-
  Bus Creator : BusCreator  Inputs=4
  Demux1 : Demux  Outputs=2
  Demux4 : Demux  Outputs=2
  Dot Product : DotProduct  InputSameDT=on  OutDataTypeStr=Inherit: Inherit via internal rule
  Gain1 : Gain  Gain=3/2/Sn
  Gain2 : Gain  Gain=3/2/Sn
  Gain3 : Gain  Gain=1/Uanp
  Gain4 : Gain  Gain=1/Iap
  Hypot : Math  Operator=hypot  RndMeth=Zero  SaturateOnIntegerOverflow=on
  Hypot1 : Math  Operator=hypot  RndMeth=Zero  SaturateOnIntegerOverflow=on
  Product3 : Product
  Product4 : Product
  pqvi : Outport
  wires:
  Gain4/1 -> Bus Creator/4  "i"
  Gain1/1 -> Bus Creator/1  "p"
  Gain2/1 -> Bus Creator/2  "q"
  Product4/1 -> Add3/2
  Dot Product/1 -> Gain1/1  "p"
  Hypot1/1 -> Gain4/1  "i"
  Gain3/1 -> Bus Creator/3  "v"
  Demux1/2 -> Hypot1/2, Product4/2
  valphabeta/1 -> Demux4/1, Dot Product/1
  Demux1/1 -> Hypot1/1, Product3/2
  ialphabeta/1 -> Demux1/1, Dot Product/2
  Add3/1 -> Gain2/1  "q"
  Demux4/2 -> Hypot/2, Product3/1
  Product3/1 -> Add3/1
  Hypot/1 -> Gain3/1  "v"
  Demux4/1 -> Hypot/1, Product4/1
  Bus Creator/1 -> pqvi/1

== matlab function PhD_Library/Adaptive Moving Averages/AMA with insertion pointer driven buffer/MATLAB Function ==
  data: x input; xavg output; n input; Nb input; xacc output; xdec output
%%%%%%%%%%%%%%%%%%%%%%%%%%%%%%%%%%%%%%%%%%%%%%%%%%%%%%%%%%%%%%%%%%%%%%%%%%
% Adaptive Moving Average Block
%%%%%%%%%%%%%%%%%%%%%%%%%%%%%%%%%%%%%%%%%%%%%%%%%%%%%%%%%%%%%%%%%%%%%%%%%%
function [xavg, xacc, xdec]  = AMAInsertionPntrDriven( x, n, Nb)

persistent buffer bufferlen rzero izero rone ione Nb_fix xavg_internal nold
 
for_acc_internal = 0;
for_dec_internal = 0;

%%%%%%%%%%%%%%%%%%%%%%%%%%%%%%%%%%
% Values of at the first cycle
%%%%%%%%%%%%%%%%%%%%%%%%%%%%%%%%%%
if isempty(buffer)
    %Nb should be larger than 2
    if Nb < 1
        %lenght of the buffer is Nb+1
        Nb_fix = 1;
        bufferlen = 2;
    else
        Nb_fix = round(Nb); %lenght of the buffer is Nb+1
        bufferlen = Nb_fix + 1;
    end
    
    %create the buffer with zeros 
    buffer = zeros(bufferlen,1);
    
    %check is n smaller or equal to Nb
    if n > Nb_fix
        n = Nb_fix;
    else
        if n < 1
            n = 1; 
        else
            n = round(n);
        end
    end
    
    %initialize pointers
    rzero = 0;
    izero = rzero + n;
    
    rone = rzero + 1;
    ione = izero + 1;
    
    %first insertion 
    %bufferlen = Nb+1 so I can write to the buffer first
    buffer(ione) = x/n;
    
    %calculating value for accumulation
    for_acc_internal = x/n;
    for_dec_internal = 0;
    
    %accumulator
    xavg_internal = for_acc_internal; 
    nold = n;
else
%%%%%%%%%%%%%%%%%%%%%%%%%%%%%%%%%%
% Here the function starts actually
%%%%%%%%%%%%%%%%%%%%%%%%%%%%%%%%%%
    %check if n smaller or equal to Nb
    if n > Nb_fix
        n = Nb_fix;
    else
        if n < 1
            n = 1; 
        else
            n = round(n);
        end
    end
    
    %insertion pointer moves forward, slot is replaced
    %bufferlen = Nb+1 so I can write to the buffer first
    izero = round( mod(izero + 1, bufferlen));
    ione = izero + 1;
    buffer(ione) = x/n;
    for_acc_internal = x/n; 
    
    %retrieval logic
    if n >= nold
        %retrieval pointer can jump backwards (as I had zeroed the buffer
        %after retrievals)
        rzero = round( mod(izero - n, bufferlen));
        rone = rzero + 1;
        for_dec_internal = buffer(rone);
        buffer(rone) = 0;
        nold = n;
    else
        jump = nold - n;
        for aux=0:jump
            rzero = round( mod(rzero + 1, bufferlen));
            rone = rzero + 1;
            for_dec_internal = for_dec_internal + buffer(rone);
            buffer(rone) = 0;
            nold = n;
        end
    end
    
    %accumulation
    xavg_internal = xavg_internal + for_acc_internal - for_dec_internal; 
end

xacc = for_acc_internal;
xdec = for_dec_internal;
xavg = xavg_internal;

== matlab function PhD_Library/Adaptive Moving Averages/AMA with retrieval pointer driven buffer/MATLAB Function ==
  data: x input; xavg output; n input; Nb input; xacc output; xdec output
%%%%%%%%%%%%%%%%%%%%%%%%%%%%%%%%%%%%%%%%%%%%%%%%%%%%%%%%%%%%%%%%%%%%%%%%%%
% Adaptive Moving Average Block
%%%%%%%%%%%%%%%%%%%%%%%%%%%%%%%%%%%%%%%%%%%%%%%%%%%%%%%%%%%%%%%%%%%%%%%%%%
% Prog/rev history
%   Mota - 2020-11-24: first release
function [xavg, xacc, xdec]  = AMARetrievalPntrDriven( x, n, Nb)

persistent buffer bufferlen r i Nb_fix xavg_internal

for_acc_internal = 0;
for_dec_internal = 0;

%%%%%%%%%%%%%%%%%%%%%%%%%%%%%%%%%%
% Values at the first cycle
%%%%%%%%%%%%%%%%%%%%%%%%%%%%%%%%%%
if isempty(buffer)
    %Nb should be larger than 1
    if Nb < 1
        %lenght of the buffer is Nb+1
        Nb_fix = 1;
        bufferlen = 2;
    else
        Nb_fix = round(Nb); %lenght of the buffer is Nb+1
        bufferlen = Nb_fix + 1;
    end
    
    %create the buffer with zeros 
    buffer = zeros(bufferlen,1);
    
    %check is n smaller or equal to Nb
    if n > Nb_fix
        n = Nb_fix;
    else
        if n < 1
            n = 1; 
        else
            n = round(n);
        end
    end
    
    %initialize pointers
    r = 1;
    i = r + n;
    
    %first sum 
    buffer(i) = buffer(i) + x/n;
    
    %calculating value for accumulation
    for_acc_internal = x/n;
    for_dec_internal = 0;
    
    %accumulator
    %xavg_internal = for_acc_internal - for_dec_internal; %first cycle, for_dec_internal=0
    xavg_internal = for_acc_internal; 
else
%%%%%%%%%%%%%%%%%%%%%%%%%%%%%%%%%%
% Here the function starts actually
%%%%%%%%%%%%%%%%%%%%%%%%%%%%%%%%%%
    %check if n smaller or equal to Nb
    if n > Nb_fix
        n = Nb_fix;
    else
        if n < 1
            n = 1; 
        else
            n = round(n);
        end
    end
    
    %pointer update
    r = r + 1;
    r = round( mod(r - 1, bufferlen) + 1); %mod works with index starting at zero, but matlab works with index on 1 
    i = round( mod(r - 1 + n, bufferlen) + 1);
    
    %insertion (sum)
    for_acc_internal = x/n; 
    buffer(i) = buffer(i) + for_acc_internal;
        
    %retrieval and zeroing 
    for_dec_internal = buffer(r);
    buffer(r) = 0; 
    
    %accumulation
    xavg_internal = xavg_internal + for_acc_internal - for_dec_internal; 
end

xacc = for_acc_internal;
xdec = for_dec_internal;
xavg = xavg_internal;

== matlab function PhD_Library/Adaptive Moving Averages/Subsystem/MATLAB Function ==
  data: x input; xavg output; xavground output; n input; Nb input; xavgceil output; xavgfloor output; xavgweigthed output; nr output; nf output; nc output; changecnt output
%%%%%%%%%%%%%%%%%%%%%%%%%%%%%%%%%%%%%%%%%%%%%%%%%%%%%%%%%%%%%%%%%%%%%%%%%%
% Adaptive Moving Average Block
%%%%%%%%%%%%%%%%%%%%%%%%%%%%%%%%%%%%%%%%%%%%%%%%%%%%%%%%%%%%%%%%%%%%%%%%%%
% Prog/rev history
%   Mota - 2020-12-08: first release

function [xavg, xavground, xavgceil, xavgfloor, xavgweigthed, nr, nf, nc, changecnt]  = AMARetrievalPntrDriven( x, n, Nb)

persistent bufferlen Nb_fix
persistent bufferround nround rround iround
persistent bufferceil nceil rceil iceil
persistent bufferfloor nfloor rfloor ifloor
persistent xavg_internal_ceil xavg_internal_round xavg_internal_floor
persistent old_nceil k_change_counter

for_acc_internal_ceil = 0;
for_dec_internal_ceil = 0;

for_acc_internal_round = 0;
for_dec_internal_round = 0;

for_acc_internal_floor = 0;
for_dec_internal_floor = 0;

nnow = n; 

%%%%%%%%%%%%%%%%%%%%%%%%%%%%%%%%%%
% Values of at the first cycle
%%%%%%%%%%%%%%%%%%%%%%%%%%%%%%%%%%
if isempty(bufferceil)
    %Nb should be larger than 1
    if Nb < 1
        %lenght of the buffer is Nb+1
        Nb_fix = 1;
        bufferlen = 2;
    else
        Nb_fix = round(Nb);%lenght of the buffer is Nb+1
        bufferlen = round(Nb_fix+1);
    end
    
    %initialize the buffer
    bufferceil = zeros(bufferlen,1);
    bufferround = zeros(bufferlen,1);
    bufferfloor = zeros(bufferlen,1);
    
    %check is n smaller or equal to Nb
    if nnow > Nb_fix
        nnow = Nb_fix;
        nceil = Nb_fix;
        nround = Nb_fix;
        nfloor = Nb_fix;
    else
        if nnow < 1
            nnow = 1;
            nceil = 1;
            nround = 1;
            nfloor = 1;
        else
            nceil = ceil(nnow);
            nround = round(nnow);
            nfloor = floor(nnow);
        end
    end
    
    %detecting change in ceiling
    old_nceil = nceil;
    k_change_counter = 0; 
    
    %initialize pointers
    rceil = 1;
    iceil = rceil + nceil;
    
    rround = 1;
    iround = rround + nround;
        
    rfloor = 1;
    ifloor = rfloor + nfloor;
        
    %first sum 
    bufferceil(iceil) = bufferceil(iceil) + x/nceil;
    bufferround(iround) = bufferround(iround) + x/nround;
    bufferfloor(ifloor) = bufferfloor(ifloor) + x/nfloor;
    
    %calculating value for accumulation
    for_acc_internal_ceil  = x/nceil;
    for_dec_internal_ceil = 0;
    
    for_acc_internal_round  = x/nround;
    for_dec_internal_round = 0;        
    
    for_acc_internal_floor  = x/nfloor;
    for_dec_internal_floor = 0;
        
    %accumulator
    xavg_internal_ceil = for_acc_internal_ceil; 
    xavg_internal_round = for_acc_internal_round; 
    xavg_internal_floor = for_acc_internal_floor; 
else
%%%%%%%%%%%%%%%%%%%%%%%%%%%%%%%%%%
% Here the function starts actually
%%%%%%%%%%%%%%%%%%%%%%%%%%%%%%%%%%
    %check is n smaller or equal to Nb
    if nnow > Nb_fix
        nnow = Nb_fix;
        nceil = Nb_fix;
        nround = Nb_fix;
        nfloor = Nb_fix;
    else
        if nnow < 1
            nnow = 1;
            nceil = 1;
            nround = 1;
            nfloor = 1;
        else
            nceil = ceil(nnow);
            nround = round(nnow);
            nfloor = floor(nnow);
        end
    end
    
    %pointer update
    %mod works from zero, matlab arrays start at index 1
    rceil = rceil + 1;
    rceil = round( mod(rceil - 1, bufferlen)+1); 
    iceil = round( mod(rceil - 1 + nceil, bufferlen) + 1);

    rround = rround + 1;
    rround = round( mod(rround - 1, bufferlen)+1); 
    iround = round( mod(rround - 1 + nround, bufferlen) + 1);
    
    rfloor = rfloor + 1;
    rfloor = round( mod(rfloor - 1, bufferlen)+1); 
    ifloor = round( mod(rfloor - 1 + nfloor, bufferlen) + 1);

    %insertion (sum)
    for_acc_internal_ceil = x/nceil; 
    bufferceil(iceil) = bufferceil(iceil) + for_acc_internal_ceil;

    for_acc_internal_round = x/nround; 
    bufferround(iround) = bufferround(iround) + for_acc_internal_round;
    
    for_acc_internal_floor = x/nfloor; 
    bufferfloor(ifloor) = bufferfloor(ifloor) + for_acc_internal_floor;

    
    %retrieval and zeroing 
    for_dec_internal_ceil = bufferceil(rceil);
    bufferceil(rceil) = 0; 

    for_dec_internal_round = bufferround(rround);
    bufferround(rround) = 0; 
        
    for_dec_internal_floor = bufferfloor(rfloor);
    bufferfloor(rfloor) = 0; 
    
    
    %accumulation
    xavg_internal_ceil = xavg_internal_ceil + for_acc_internal_ceil - for_dec_internal_ceil; 
    xavg_internal_round = xavg_internal_round + for_acc_internal_round - for_dec_internal_round; 
    xavg_internal_floor = xavg_internal_floor + for_acc_internal_floor - for_dec_internal_floor; 
end

xavgceil = xavg_internal_ceil;
xavground = xavg_internal_round;
xavgfloor = xavg_internal_floor;
xavgweigthed = (nnow - nfloor) * xavg_internal_ceil + (1 - nnow + nfloor) * xavg_internal_floor;
%alpha = (nnow - nfloor);
%oneminusalpha = (1 - nnow + nfloor);

nr = nround;
nf = nfloor;
nc = nceil;
changenc = 0;

%Check for changes in nceil and start a timer
if old_nceil ~= nceil
    changenc = 1;
    k_change_counter = 1; 
else
    if k_change_counter > 0
        k_change_counter = k_change_counter  + 1;
        if k_change_counter > nceil
            changenc = 0; 
            k_change_counter = 0;
        else
            changenc = 1;
        end
    end
end

if changenc == 1
    xavg = xavg_internal_round;
else
    xavg = (nnow - nfloor) * xavg_internal_ceil + (1 - nnow + nfloor) * xavg_internal_floor;
end
old_nceil = nceil;
changecnt = k_change_counter;

== matlab function PhD_Library/Offshore_Oil_and_Wind/idqref_gen_for_cnst_p/MATLAB Function ==
  data: vdqp input; idqref output; vdqn input; idqref input
function idqref = fcn(vdqp,vdqn,idqref)

% Calculation of the negative sequence references for zeroing the active 
% power second harmonic oscillations
% 
% Derived independently from, but later noticed that the same line of
% reasoning was adopted by Chaudhary 2012 "Negative Sequence Current
% Control in Wind Power Plants With VSC-HVDC Connection"

% In "expanded" matrix form
% | idn | = - | -vdp  +vqp |^{-1} * | -vdn  +vqn | * | idp | 
% | iqn | =   | +vqp  +vdp |        | -vdn  +vqn |   | idq |
% In matrix form
%  idqn   = -   vdqp^{-1}         *      vdqn      *   idqp

%The matrix that will be inverted
vp = zeros(2);
vp(1,1) = -vdqp(1);
vp(1,2) = vdqp(2);
vp(2,1) = vdqp(2);
vp(2,2) = vdqp(1);

%check is vp is invertible
if det(vp) == 0
    idqref(1,1) = 0;
    idqref(2,1) = 0;
else
    %The matrix that is not inverted
    vn = zeros(2);
    vn(1,1) = -vdqn(1);
    vn(1,2) = vdqn(2);
    vn(2,1) = vdqn(2);
    vn(2,2) = vdqn(1);

    % idqn = - vdqp^{-1} * vdqn * idqp
    idqref = -vp\vn*idqref;
end

== matlab function PhD_Library/Offshore_Oil_and_Wind/digital_integrator/MATLAB Function ==
  data: x input; y output; max input; min input; force input; forceval input; Ts input
%%%%%%%%%%%%%%%%%%%%%%%%%%%%%%%%%%%%%%%%%%%%%%%%%%%%%%%%%%%%%%%%%%%%%%%%%%
% Digital integrator
%%%%%%%%%%%%%%%%%%%%%%%%%%%%%%%%%%%%%%%%%%%%%%%%%%%%%%%%%%%%%%%%%%%%%%%%%%\
% Forward Euler method: as in matlab help
%   y(n) = y(n-1) + Ts(n-1)*x(n-1)
%   uset it to avoid algebraic loops

% All inputs are stored in states, so there is no direct feedthrough
% GAMBIARRA for avoiding algebraic loops
% see: https://www.mathworks.com/help/simulink/ug/integration-considerations-for-matlab-function-blocks.html

% Inputs
%   x: input to the integrator
%   max: max value for integrator
%   min: min value for integrator
%   force: if=1 sets integrator to forceval
%   forceval: see line above (max and min are respected
%   Ts: sampling time
% Output
%   y: output of the integrator

%%%%%%%%%%%%%%%%%%%%%%%%%%%%%%%%%%%%%%%%%%%%%%%%%%%%%%%%%%%%%%%%%%%%%%%%%%\
% Prog/rev history
%   Mota - 2021-05-21: first release

function y = DigInt(x, max, min, force, forceval, Ts)

% The value of the integrator
persistent i
persistent old_x
persistent old_max
persistent old_min
persistent old_force
persistent old_forceval
persistent old_Ts

% Only at first cycle - outputs zero
if isempty(i)
    y = 0;
    i = 0;
    old_x = 0;
    old_max = 0;
    old_min = 0;
    old_force = 0;
    old_forceval = 0;
    old_Ts = 0;
    % On the second cycle, output will still be zero, due to choices above
    return;
end

% auxiliary value
aux = 0;

% Bypassing the integrator with a value (can be used for followup)
if old_force >= 1
    aux = old_forceval;
else
    %if not bypass, then calculate the next value of the integrator
    aux = i + old_Ts*old_x;
end

%Limiting the integrator
if aux > old_max
    % max value has priority, i.e.,
    % if "max" is below "min" due to engineer error
    % the integrator will stop at "max"
    aux = old_max;
elseif aux < old_min
    % if integrator would cross the min, it will be stopped at min
    aux = old_min;
end

% output of the integrator
y = aux;

%update states
i = aux;
old_x = x;
old_max = max;
old_min = min;
old_force = force;
old_forceval = forceval;
old_Ts = Ts;
